simulink model "testGravityTorque"  (R2021a)
settings: Solver=VariableStepAuto  StartTime=0.0  StopTime=Torb  RelTol=1e-3
libraries: sharedtransform x1
settings Model: DataDictionary=databus.sldd  Creator=Laura  LastModifiedBy=Laura

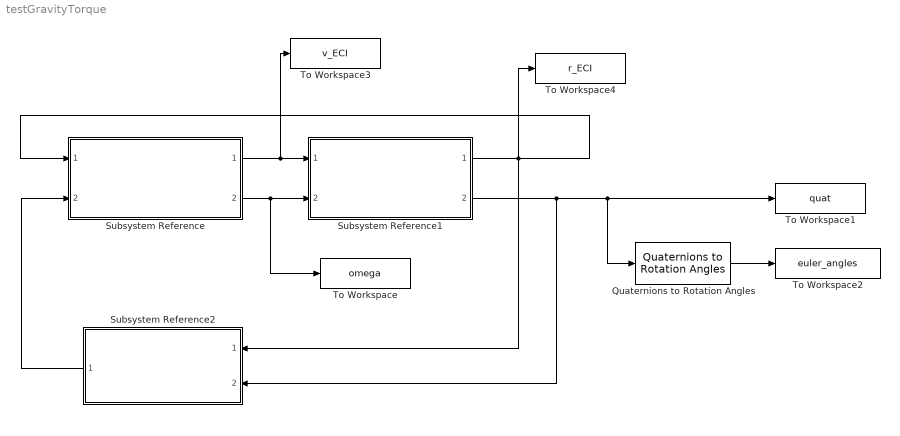
== system testGravityTorque ==
  Quaternions to Rotation Angles : sharedtransform/Quaternions to Rotation Angles  rotationOrder=ZYX  aMode=aMode
      settings: SourceProductBaseCode=AE,PW,DR,MT,UV,VE
  Subsystem Reference : Subsystem  ReferencedSubsystem=Dynamics
  Subsystem Reference1 : Subsystem  ReferencedSubsystem=Kinematics
  Subsystem Reference2 : Subsystem  ReferencedSubsystem=GravityTorque
  To Workspace : ToWorkspace  VariableName=omega  SaveFormat=Timeseries  SampleTime=-1
  To Workspace1 : ToWorkspace  VariableName=quat  SaveFormat=Timeseries  SampleTime=-1
  To Workspace2 : ToWorkspace  VariableName=euler_angles  SaveFormat=Timeseries  SampleTime=-1
  To Workspace3 : ToWorkspace  VariableName=v_ECI  SaveFormat=Timeseries  SampleTime=-1
  To Workspace4 : ToWorkspace  VariableName=r_ECI  SaveFormat=Timeseries  SampleTime=-1
  wires:
  Subsystem Reference2/1 -> Subsystem Reference/2
  Subsystem Reference1/1 -> To Workspace4/1, Subsystem Reference2/1, Subsystem Reference/1
  Subsystem Reference1/2 -> Subsystem Reference2/2, To Workspace1/1, Quaternions to Rotation Angles/1
  Subsystem Reference/2 -> To Workspace/1, Subsystem Reference1/2
  Subsystem Reference/1 -> To Workspace3/1, Subsystem Reference1/1
  Quaternions to Rotation Angles/1 -> To Workspace2/1
